simulink library "mbd_s32k1xx_ec_toolbox"  (Simulink 9.0)
settings: Solver=FixedStepDiscrete  StartTime=0.0  StopTime=10.0  FixedStep=0.1  RelTol=1e-3  EnableMultiTasking=on
InitFcn:
  | mbd_s32k_consistency_checks(bdroot(gcs));
(part 3 of 8)

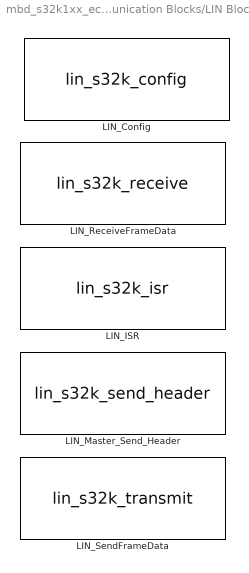
== system mbd_s32k1xx_ec_toolbox/Communication Blocks/LIN Blocks ==
  LIN_Config : S-Function  FunctionName=lin_s32k_config  SFunctionDeploymentMode=off  EnableBusSupport=off  mask(lin_s32k_config){instance=2, baudrate=9600, node_function=MASTER, autobaud_enable=None, rx=PTD6: [LPUART2_RX | Receive], tx=PTD7: [LPUART2_TX | Transmit], cts=PTC12: [LPUART2_CTS | Clear To Send (bar)], rts=PTC13: [LPUART2_RTS | Request To Send]}
      mask prompts: instance "LIN"; baudrate "Baud rate"; node_function "Node function"; autobaud_enable "Autobaud"
      mask help: This block allows to configure LIN module.
      mask init:
      | maskStr = mbd_s32k_lin_config_init();
      | mbd_s32k_lpuart_display_instances(gcb, 'instance');
      | mbd_s32k_lpuart_instance_callback(gcb);
      settings: NameChangeFcn=mbd_s32k_name_check(gcb);
      mask Help: web(fullfile(mbd_s32k_block_help, 'lin', 'lin_config.html'));
      mask TypeOptions instance: 0 | 1 | 2
      mask Callback instance:
      | mbd_s32k_lpuart_instance_callback(gcb);
      | mbd_s32k_lpuart_display_instances(gcb, 'instance');
      mask TypeOptions baudrate: 1200 | 2400 | 4800 | 9600 | 14400 | 19200 | 38400 | 56000 | 57600 | 115200 | 128000 | 256000
      mask TypeOptions node_function: MASTER | SLAVE
      mask TypeOptions autobaud_enable: None | Even | Odd
      mask TypeOptions rx: PTA8: [LPUART2_RX | Receive] | PTA30: [LPUART2_RX | Receive] | PTD6: [LPUART2_RX | Receive] | PTD17: [LPUART2_RX | Receive]
      mask TypeOptions tx: PTA9: [LPUART2_TX | Transmit] | PTA29: [LPUART2_TX | Transmit] | PTD7: [LPUART2_TX | Transmit] | PTE12: [LPUART2_TX | Transmit]
      mask TypeOptions cts: PTC12: [LPUART2_CTS | Clear To Send (bar)] | PTD11: [LPUART2_CTS | Clear To Send (bar)] | PTE9: [LPUART2_CTS | Clear To Send (bar)]
      mask TypeOptions rts: PTC13: [LPUART2_RTS | Request To Send] | PTD12: [LPUART2_RTS | Request To Send] | PTE3: [LPUART2_RTS | Request To Send]
      mask Display:
      | disp(maskStr);
      | image('nxp_logo.png', 'top-right');
  LIN_ISR : S-Function  FunctionName=lin_s32k_isr  Parameters=out_array  SFunctionDeploymentMode=off  EnableBusSupport=off  mask(lin_s32k_isr){instance=2}
      mask prompts: instance "LPUART"
      mask help: This block allows to create receive/transmit ISR routine for the LIN module.
      mask init:
      | mbd_s32k_lpuart_display_instances(gcb, 'instance');
      | [out_struct, out_array] = mbd_s32k_lin_isr_info(gcb);
      | maskStr = mbd_s32k_lin_isr_string();
      settings: NameChangeFcn=mbd_s32k_name_check(gcb);
      mask Help: web(fullfile(mbd_s32k_block_help, 'lin', 'lin_isr.html'));
      mask TypeOptions instance: 0 | 1 | 2
      mask Callback instance: mbd_s32k_lpuart_display_instances(gcb, 'instance');
      mask Display:
      | port_label('output',1,'Trigger')
      | port_label('output',2,'Event')
      | port_label('output',3,'FrameID')
      | disp(maskStr);
      | image('nxp_logo.png', 'top-right');
  LIN_Master_Send_Header : S-Function  FunctionName=lin_s32k_send_header  Parameters=instance  SFunctionDeploymentMode=off  EnableBusSupport=off  mask(lin_s32k_send_header){instance=2}
      mask prompts: instance "LPUART"
      mask help: This block allows to send header [only in master mode].
      mask init:
      | mbd_s32k_lpuart_display_instances(gcb, 'instance');
      settings: NameChangeFcn=mbd_s32k_name_check(gcb);
      mask Help: web(fullfile(mbd_s32k_block_help, 'lin', 'lin_master_send_header.html'));
      mask TypeOptions instance: 0 | 1 | 2
      mask Callback instance: mbd_s32k_lpuart_display_instances(gcb, 'instance');
      mask Display:
      | disp(['LIN ', get_param(gcb, 'instance')]);
      | port_label('input',1,'ID');
      | image('nxp_logo.png', 'top-right');
  LIN_ReceiveFrameData : S-Function  FunctionName=lin_s32k_receive  SFunctionDeploymentMode=off  EnableBusSupport=off  mask(lin_s32k_receive_data){instance=2}
      mask prompts: instance "LIN"
      mask help: This block allows to read data received on LIN bus.
      mask init:
      | mbd_s32k_lpuart_display_instances(gcb, 'instance');
      settings: NameChangeFcn=mbd_s32k_name_check(gcb);
      mask Help: web(fullfile(mbd_s32k_block_help, 'lin', 'lin_receive_frame_data.html'));
      mask TypeOptions instance: 0 | 1 | 2
      mask Callback instance: mbd_s32k_lpuart_display_instances(gcb, 'instance');
      mask Display:
      | disp(['LIN ', get_param(gcb, 'instance')]);
      | port_label('output',1,'data');
      | port_label('input',1,'size');
      | image('nxp_logo.png', 'top-right');
  LIN_SendFrameData : S-Function  FunctionName=lin_s32k_transmit  Parameters=instance  SFunctionDeploymentMode=off  EnableBusSupport=off  mask(lin_s32k_transmit_data){instance=2}
      mask prompts: instance "LPUART"
      mask help: This block allows to transmit data via LIN.
      mask init:
      | mbd_s32k_lpuart_display_instances(gcb, 'instance');
      settings: NameChangeFcn=mbd_s32k_name_check(gcb);
      mask Help: web(fullfile(mbd_s32k_block_help, 'lin', 'lin_send_frame_data.html'));
      mask TypeOptions instance: 0 | 1 | 2
      mask Callback instance: mbd_s32k_lpuart_display_instances(gcb, 'instance');
      mask Display:
      | disp(['LIN ', get_param(gcb, 'instance')]);
      | port_label('input',1,'data');
      | image('nxp_logo.png', 'top-right');

== system mbd_s32k1xx_ec_toolbox/Communication Blocks/SPI Blocks ==
  "LPSPI_Config " : S-Function  FunctionName=lpspi_s32k_config  SFunctionDeploymentMode=off  EnableBusSupport=off  mask(lpspi_s32k_config){InstanceNumber=0, Role=Master, BaudRate=10000, ShowAdvanced=on, sin=PTB3: [LPSPI0_SIN | LPSPI Serial Data Input], sout=PTB1: [LPSPI0_SOUT | LPSPI Serial Data Output], sck=PTB2: [LPSPI0_SCK | LPSPI Serial Clock I/O], pcs0=PTB0: [LPSPI0_PCS0 | Peripheral Chip Select 0], pcs1=PTB5: [LPSPI0_PCS1 | Peripheral Chip Select 1], pcs2=PTE6: [LPSPI0_PCS2 | Peripheral Chip Select 2], pcs3=PTA15: [LPSPI0_PCS3 | Peripheral Chip Select 3], CPHA=0, CPOL=0, BitOrder=MSB first, TransferSize=8, WhichPCS=0, PCSPol=ActiveLow, ContinuousTransfer=off}
      mask prompts: InstanceNumber "Instance"; BaudRate "Baud Rate, bps"; ShowAdvanced "Show advanced options"; BitOrder "Bit order"; TransferSize "Frame size"; WhichPCS "Peripheral CS"; PCSPol "Peripheral CS Polarity"; ContinuousTransfer "Continuous Transfer"
      mask help: This block allows to configure LPSPI module.
      mask init:
      | maskStr = mbd_s32k_lpspi_config_string();
      | mbd_s32k_lpspi_display_instances();
      settings: NameChangeFcn=mbd_s32k_name_check(gcb);
      mask Help: web(fullfile(mbd_s32k_block_help, 'lpspi', 'lpspi_config.html'));
      mask TypeOptions InstanceNumber: 0 | 1 | 2
      mask Callback InstanceNumber:
      | mbd_s32k_lpspi_instance_callback(gcb);
      | mbd_s32k_lpspi_display_instances();
      mask TypeOptions Role: Master | Slave
      mask Callback Role: mbd_s32k_lpspi_config_cbk
      mask Callback ShowAdvanced: mbd_s32k_lpspi_config_cbk()
      mask TypeOptions sin: PTB3: [LPSPI0_SIN | LPSPI Serial Data Input] | PTD16: [LPSPI0_SIN | LPSPI Serial Data Input] | PTE1: [LPSPI0_SIN | LPSPI Serial Data Input]
      mask TypeOptions sout: PTA30: [LPSPI0_SOUT | LPSPI Serial Data Output] | PTB1: [LPSPI0_SOUT | LPSPI Serial Data Output] | PTB4: [LPSPI0_SOUT | LPSPI Serial Data Output] | PTE2: [LPSPI0_SOUT | LPSPI Serial Data Output]
      mask TypeOptions sck: PTB2: [LPSPI0_SCK | LPSPI Serial Clock I/O] | PTC23: [LPSPI0_SCK | LPSPI Serial Clock I/O] | PTD15: [LPSPI0_SCK | LPSPI Serial Clock I/O] | PTE0: [LPSPI0_SCK | LPSPI Serial Clock I/O]
      mask TypeOptions pcs0: None | PTA26: [LPSPI0_PCS0 | Peripheral Chip Select 0] | PTB0: [LPSPI0_PCS0 | Peripheral Chip Select 0] | PTB5: [LPSPI0_PCS0 | Peripheral Chip Select 0]
      mask TypeOptions pcs1: None | PTA31: [LPSPI0_PCS1 | Peripheral Chip Select 1] | PTB5: [LPSPI0_PCS1 | Peripheral Chip Select 1]
      mask TypeOptions pcs2: None | PTE6: [LPSPI0_PCS2 | Peripheral Chip Select 2]
      mask TypeOptions pcs3: None | PTA15: [LPSPI0_PCS3 | Peripheral Chip Select 3]
      mask TypeOptions CPHA: 0 | 1
      mask TypeOptions CPOL: 0 | 1
      mask TypeOptions BitOrder: MSB first | LSB first
      mask TypeOptions WhichPCS: 0 | 1 | 2 | 3
      mask TypeOptions PCSPol: ActiveLow | ActiveHigh
      mask Display:
      | disp(maskStr);
      | image('nxp_logo.png', 'top-right');
  LPSPI_ISR : S-Function  FunctionName=lpspi_s32k_isr  SFunctionDeploymentMode=off  EnableBusSupport=off  mask(lpspi_s32k_isr){instanceNumber=0, isr_lvl=0, role=Master, transfer_end=off, spi_upd=on}
      mask prompts: instanceNumber "Instance"; isr_lvl "ISR Level"; transfer_end "Transfer END"
      mask help: This block allows to create ISR routine (only callback at END OF TRANSFER event) for the LPSPI module.
      mask init:
      | maskStr = mbd_s32k_lpspi_isr_string(gcb);
      settings: NameChangeFcn=mbd_s32k_name_check(gcb);
      mask Help: web(fullfile(mbd_s32k_block_help, 'lpspi', 'lpspi_isr.html'));
      mask TypeOptions instanceNumber: 0 | 1 | 2
      mask TypeOptions isr_lvl: 0 | 1 | 2 | 3 | 4 | 5 | 6 | 7 | 8 | 9 | 10 | 11 | 12 | 13 | 14 | 15
      mask TypeOptions role: Master | Slave
      mask Display:
      | port_label('output',1,'Trigger')
      | disp(maskStr);
      | image('nxp_logo.png', 'top-right');
  LPSPI_Master_Transfer : S-Function  FunctionName=lpspi_s32k_master_transfer  Parameters=instance  SFunctionDeploymentMode=off  EnableBusSupport=off  mask(lpspi_s32k_master_transfer){instance=0, pcs=0, pcs_polarity=ActiveLow, xfermode=Non blocking, timeout=50, spi_upd=on}
      mask prompts: pcs_polarity "PCS Polarity"; xfermode "Transfer mode"
      mask help: Allows to transmit data through a SPI module.
      mask init:
      | maskStr = mbd_s32k_lpspi_master_tx_string(gcb);
      settings: NameChangeFcn=mbd_s32k_name_check(gcb);
      mask Help: web(fullfile(mbd_s32k_block_help, 'lpspi', 'lpspi_master_transfer.html'));
      mask TypeOptions instance: 0 | 1 | 2
      mask TypeOptions pcs: 0 | 1 | 2 | 3
      mask TypeOptions pcs_polarity: ActiveLow | ActiveHigh
      mask TypeOptions xfermode: Blocking | Non blocking
      mask Callback xfermode: mbd_s32k_lpspi_transfer_cbk
      mask Display:
      | port_label('input',1,'Data Tx')
      | port_label('output',1,'Data Rx')
      | disp(maskStr);
      | image('nxp_logo.png', 'top-right');
  LPSPI_Slave_Transfer : S-Function  FunctionName=lpspi_s32k_slave_transfer  Parameters=instance  SFunctionDeploymentMode=off  EnableBusSupport=off  mask(lpspi_s32k_slave_transfer){instance=0, pcs=0, pcs_polarity=ActiveLow, xfermode=Non blocking, timeout=50, spi_upd=on}
      mask prompts: pcs_polarity "PCS Polarity"; xfermode "Transfer mode"
      mask help: Allows to transmit data through a SPI module.
      mask init:
      | maskStr = mbd_s32k_lpspi_master_tx_string(gcb);
      settings: NameChangeFcn=mbd_s32k_name_check(gcb);
      mask Help: web(fullfile(mbd_s32k_block_help, 'lpspi', 'lpspi_slave_transfer.html'));
      mask TypeOptions instance: 0 | 1 | 2
      mask TypeOptions pcs: 0 | 1 | 2 | 3
      mask TypeOptions pcs_polarity: ActiveLow | ActiveHigh
      mask TypeOptions xfermode: Blocking | Non blocking
      mask Callback xfermode: mbd_s32k_lpspi_transfer_cbk
      mask Display:
      | port_label('input',1,'Data Tx')
      | port_label('output',1,'Data Rx')
      | disp(maskStr);
      | image('nxp_logo.png', 'top-right');

== system mbd_s32k1xx_ec_toolbox/Communication Blocks/UART Blocks ==
  LPUART_Config : S-Function  FunctionName=lpuart_s32k_config  SFunctionDeploymentMode=off  EnableBusSupport=off  mask(lpuart_s32k_config){instance=0, baudrate=115200, databits=8, parity=None, sbns=1, bothedge=rising edge, rxinv=off, txinv=off, show_adv_opts=on, brk13=10 - 13 bit times, lbkde=10 - 13 bit times, rx=PTA2: [LPUART0_RX | Receive], tx=PTA3: [LPUART0_TX | Transmit], cts=PTA0: [LPUART0_CTS | Clear To Send (bar)], rts=PTA1: [LPUART0_RTS | Request To Send]}
      mask prompts: instance "LPUART"; baudrate "Baud rate"; databits "Data bits"; parity "Parity mode"; sbns "Stop bit number select"; bothedge "Both edge sampling"; rxinv "Receive data inversion"; txinv "Transmit data inversion"; show_adv_opts "Show advanced options"; brk13 "Transmit break character length"; lbkde "Receive break character detection length"
      mask help: This block allows to configure LPUART module.
      mask init:
      | maskStr = mbd_s32k_lpuart_config_init();
      | mbd_s32k_lpuart_display_instances(gcb, 'instance');
      | mbd_s32k_lpuart_instance_callback(gcb);
      settings: NameChangeFcn=mbd_s32k_name_check(gcb);
      mask Help: web(fullfile(mbd_s32k_block_help, 'lpuart', 'lpuart_config.html'));
      mask TypeOptions instance: 0 | 1 | 2
      mask Callback instance:
      | mbd_s32k_lpuart_instance_callback(gcb);
      | mbd_s32k_lpuart_display_instances(gcb, 'instance');
      mask TypeOptions baudrate: 1200 | 2400 | 4800 | 9600 | 14400 | 19200 | 38400 | 56000 | 57600 | 115200 | 128000 | 256000
      mask TypeOptions databits: 8 | 9 | 10
      mask TypeOptions parity: None | Even | Odd
      mask TypeOptions sbns: 1 | 2
      mask TypeOptions bothedge: rising edge | rising and falling edges
      mask Callback show_adv_opts: mbd_s32k_lpuart_config_cbk()
      mask TypeOptions brk13: 10 - 13 bit times | 13 - 16 bit times
      mask TypeOptions lbkde: 10 - 13 bit times | 13 - 16 bit times
      mask TypeOptions rx: PTA2: [LPUART0_RX | Receive] | PTA28: [LPUART0_RX | Receive] | PTB0: [LPUART0_RX | Receive] | PTC2: [LPUART0_RX | Receive]
      mask TypeOptions tx: PTA3: [LPUART0_TX | Transmit] | PTA27: [LPUART0_TX | Transmit] | PTB1: [LPUART0_TX | Transmit] | PTC3: [LPUART0_TX | Transmit]
      mask TypeOptions cts: PTA0: [LPUART0_CTS | Clear To Send (bar)] | PTC8: [LPUART0_CTS | Clear To Send (bar)]
      mask TypeOptions rts: PTA1: [LPUART0_RTS | Request To Send] | PTC9: [LPUART0_RTS | Request To Send]
      mask Display:
      | image('nxp_logo.png', 'top-right');
      | disp(maskStr);
  LPUART_Receive : S-Function  FunctionName=lpuart_s32k_receive  SFunctionDeploymentMode=off  EnableBusSupport=off  mask(lpuart_s32k_receive){instance=0}
      mask prompts: instance "LPUART"
      mask help: This block allows to read data from LPUART.
      mask init:
      | mbd_s32k_lpuart_display_instances(gcb, 'instance');
      settings: NameChangeFcn=mbd_s32k_name_check(gcb);
      mask Help: web(fullfile(mbd_s32k_block_help, 'lpuart', 'lpuart_receive.html'));
      mask TypeOptions instance: 0 | 1 | 2
      mask Callback instance: mbd_s32k_lpuart_display_instances(gcb, 'instance');
      mask Display:
      | image('nxp_logo.png', 'top-right');
      | disp(['LPUART', get_param(gcb, 'instance')]);
      | port_label('output',1,'data');
      | port_label('input',1,'size');
  LPUART_RxTx_ISR : S-Function  FunctionName=lpuart_s32k_rxtx_isr  Parameters=out_array  SFunctionDeploymentMode=off  EnableBusSupport=off  mask(lpuart_s32k_rxtx_isr){instance=0, prio=0, tie=off, tcie=off, rie=off, ilie=off}
      mask prompts: instance "LPUART"; prio "ISR Priority"; tie "Transmit buffer empty"; tcie "End of transfer"; rie "Receiver buffer full"; ilie "Error event"
      mask help: This block allows to create receive/transmit ISR routine for the LPUART module.
      mask init:
      | mbd_s32k_lpuart_display_instances(gcb, 'instance');
      | [out_struct, out_array] = mbd_s32k_lpuart_isr_info(gcb);
      | maskStr = mbd_s32k_lpuart_isr_string();
      settings: NameChangeFcn=mbd_s32k_name_check(gcb);
      mask Help: web(fullfile(mbd_s32k_block_help, 'lpuart', 'lpuart_rxtx_isr.html'));
      mask TypeOptions instance: 0 | 1 | 2
      mask Callback instance: mbd_s32k_lpuart_display_instances(gcb, 'instance');
      mask TypeOptions prio: 0 | 1 | 2 | 3 | 4 | 5 | 6 | 7 | 8 | 9 | 10 | 11 | 12 | 13 | 14 | 15
      mask Callback prio: mbd_s32k_isr_priority_cbk(gcb, 'prio')
      mask Display:
      | image('nxp_logo.png', 'top-right');
      | port_label('output',1,'Trigger')
      | port_label('output',2,'Status')
      | disp(maskStr);
  LPUART_Transmit : S-Function  FunctionName=lpuart_s32k_transmit  SFunctionDeploymentMode=off  EnableBusSupport=off  mask(lpuart_s32k_transmit){instance=0}
      mask prompts: instance "LPUART"
      mask help: This block allows to transmit data via LPUART.
      mask init:
      | mbd_s32k_lpuart_display_instances(gcb, 'instance');
      settings: NameChangeFcn=mbd_s32k_name_check(gcb);
      mask Help: web(fullfile(mbd_s32k_block_help, 'lpuart', 'lpuart_transmit.html'));
      mask TypeOptions instance: 0 | 1 | 2
      mask Callback instance: mbd_s32k_lpuart_display_instances(gcb, 'instance');
      mask Display:
      | image('nxp_logo.png', 'top-right');
      | disp(['LPUART', get_param(gcb, 'instance')]);
      | port_label('input',1,'data')

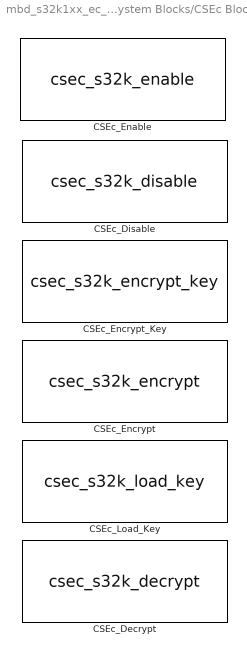
== system mbd_s32k1xx_ec_toolbox/Core and System Blocks/CSEc Blocks ==
  CSEc_Decrypt : S-Function  FunctionName=csec_s32k_decrypt  Parameters=sFuncParams  SFunctionDeploymentMode=off  EnableBusSupport=off  mask(csec_s32k_decrypt){csec_mode=Electronic Codebook (ECB), csec_key_id=RAM_KEY, csec_timeout=1}
      mask prompts: csec_mode "Mode"; csec_key_id "Key ID"; csec_timeout "Timeout (ms)"
      mask help: This block allows to decrypt a cipher text.
      mask init:
      | crlf = sprintf('\n');
      | 
      | mode = get_param(gcb, 'csec_mode');
      | keyId = get_param(gcb, 'csec_key_id');
      | 
      | startIdx = strfind(mode, '(') + 1;
      | endIdx = length(mode) - 1;
      | mode = mode(startIdx:endIdx);
      | 
      | maskStr = [
      |     'CSEc Decrypt' crlf ...
      |     crlf ...
      |     'Mode: ' mode crlf ...
      |     'Key ID: ' keyId crlf];
      | 
      | maskStr = mbd_s32k_csec_init(maskStr);
      | 
      | sFuncParams = uint32([csec_mode])';
      settings: NameChangeFcn=mbd_s32k_name_check(gcb);
      mask Help: web(fullfile(mbd_s32k_block_help, 'csec', 'csec_decrypt.html'));
      mask TypeOptions csec_mode: Electronic Codebook (ECB) | Cipher Block Chaining (CBC)
      mask TypeOptions csec_key_id: RAM_KEY | KEY_1 | KEY_2 | KEY_3 | KEY_4 | KEY_5 | KEY_6 | KEY_7 | KEY_8 | KEY_9 | KEY_10 | KEY_11 | KEY_12 | KEY_13 | KEY_14 | KEY_15 | KEY_16 | KEY_17
      mask Callback csec_timeout: mbd_s32k_csec_decrypt_cbk('csec_timeout');
      mask DialogControl ParametersGroupbox Prompt: Parameters
      mask Display:
      | disp(maskStr);
      | 
      | mode = get_param(gcb, 'csec_mode');
      | 
      | port_label('input', 1, 'Cipher text');
      | if strcmp(mode, 'Cipher Block Chaining (CBC)')
      |     port_label('input', 2, 'IV');
      | end
      | 
      | port_label('output', 1, 'Status');
      | port_label('output', 2, 'Plain text');
      | 
      | image('nxp_logo.png', 'top-right');
  CSEc_Disable : S-Function  FunctionName=csec_s32k_disable  Parameters=sFuncParams  SFunctionDeploymentMode=off  EnableBusSupport=off  mask(csec_s32k_disable){csec_master_key={'0xff', '0xff', '0xff', '0xff', '0xff', '0xff', '0xff', '0xff', '0xff', '0xff', '0xff', '0xff', '0xff', '0xff', '0xff', '0xff'}}
      mask prompts: csec_master_key "Master key"
      mask help: This block allows to disable the CSEc module.
      mask init:
      | maskStr = mbd_s32k_csec_init('CSec Disable');
      | 
      | sFuncParams = uint32([])';
      settings: NameChangeFcn=mbd_s32k_name_check(gcb);
      mask Help: web(fullfile(mbd_s32k_block_help, 'csec', 'csec_disable.html'));
      mask Display:
      | disp(maskStr);
      | port_label('output', 1, 'Status');
      | image('nxp_logo.png', 'top-right');
  CSEc_Enable : S-Function  FunctionName=csec_s32k_enable  Parameters=sFuncParams  SFunctionDeploymentMode=off  EnableBusSupport=off  mask(csec_s32k_enable){csec_num_user_keys=20 keys}
      mask prompts: csec_num_user_keys "User keys"
      mask help: This block allows to enable the CSEc module.
      mask init:
      | maskStr = mbd_s32k_csec_init('CSEc Enable');
      | 
      | sFuncParams = uint32([])';
      settings: NameChangeFcn=mbd_s32k_name_check(gcb);
      mask Help: web(fullfile(mbd_s32k_block_help, 'csec', 'csec_enable.html'));
      mask TypeOptions csec_num_user_keys: Zero | 5 keys | 10 keys | 20 keys
      mask Display:
      | disp(maskStr);
      | image('nxp_logo.png', 'top-right');
  CSEc_Encrypt : S-Function  FunctionName=csec_s32k_encrypt  Parameters=sFuncParams  SFunctionDeploymentMode=off  EnableBusSupport=off  mask(csec_s32k_encrypt){csec_mode=Electronic Codebook (ECB), csec_key_id=RAM_KEY, csec_timeout=1}
      mask prompts: csec_mode "Mode"; csec_key_id "Key ID"; csec_timeout "Timeout (ms)"
      mask help: This block allows to encrypt a plain text.
      mask init:
      | crlf = sprintf('\n');
      | 
      | mode = get_param(gcb, 'csec_mode');
      | keyId = get_param(gcb, 'csec_key_id');
      | 
      | startIdx = strfind(mode, '(') + 1;
      | endIdx = length(mode) - 1;
      | mode = mode(startIdx:endIdx);
      | 
      | 
      | maskStr = [
      |     'CSEc Encrypt' crlf ...
      |     crlf ...
      |     'Mode: ' mode crlf ...
      |     'Key ID: ' keyId crlf];
      | 
      | maskStr = mbd_s32k_csec_init(maskStr);
      | 
      | sFuncParams = uint32([csec_mode])';
      settings: NameChangeFcn=mbd_s32k_name_check(gcb);
      mask Help: web(fullfile(mbd_s32k_block_help, 'csec', 'csec_encrypt.html'));
      mask TypeOptions csec_mode: Electronic Codebook (ECB) | Cipher Block Chaining (CBC)
      mask TypeOptions csec_key_id: RAM_KEY | KEY_1 | KEY_2 | KEY_3 | KEY_4 | KEY_5 | KEY_6 | KEY_7 | KEY_8 | KEY_9 | KEY_10 | KEY_11 | KEY_12 | KEY_13 | KEY_14 | KEY_15 | KEY_16 | KEY_17
      mask Callback csec_timeout: mbd_s32k_csec_encrypt_cbk('csec_timeout');
      mask Display:
      | disp(maskStr);
      | 
      | mode = get_param(gcb, 'csec_mode');
      | 
      | port_label('input', 1, 'Plain text');
      | if strcmp(mode, 'Cipher Block Chaining (CBC)')
      |     port_label('input', 2, 'IV');
      | end
      | 
      | port_label('output', 1, 'Status');
      | port_label('output', 2, 'Cipher text');
      | 
      | image('nxp_logo.png', 'top-right');
  CSEc_Encrypt_Key : S-Function  FunctionName=csec_s32k_encrypt_key  Parameters=[]  SFunctionDeploymentMode=off  EnableBusSupport=off  mask(csec_s32k_encrypt_key){csec_key_id=MASTER_ECU, csec_key={'0xff', '0xff', '0xff', '0xff', '0xff', '0xff', '0xff', '0xff', '0xff', '0xff', '0xff', '0xff', '0xff', '0xff', '0xff', '0xff'}, csec_auth_key_id=MASTER_ECU, csec_auth_key={'0xff', '0xff', '0xff', '0xff', '0xff', '0xff', '0xff', '0xff', '0xff', '0xff', '0xff', '0xff', '0xff', '0xff', '0xff', '0xff'}, csec_counter=1}
      mask prompts: csec_key_id "Key ID"; csec_key "Key"; csec_auth_key_id "Auth key ID"; csec_auth_key "Auth key"; csec_counter "Counter (28 bits)"
      mask help: This block allows to encrypt the key before loading it into CSEc module.
      mask init:
      | crlf = sprintf('\n');
      | 
      | authKeyId = get_param(gcb, 'csec_auth_key_id');
      | keyId = get_param(gcb, 'csec_key_id');
      | 
      | maskStr = [
      |     'CSEc Encrypt Key' crlf ...
      |     crlf ...
      |     'Key ID : ' keyId crlf ...
      |     'Authorization Key ID : ' authKeyId crlf];
      | 
      | maskStr = mbd_s32k_csec_init(maskStr);
      | 
      | sFuncParams = uint32([])';
      settings: NameChangeFcn=mbd_s32k_name_check(gcb);
      mask Help: web(fullfile(mbd_s32k_block_help, 'csec', 'csec_encrypt_key.html'));
      mask TypeOptions csec_key_id: MASTER_ECU | RAM_KEY | KEY_1 | KEY_2 | KEY_3 | KEY_4 | KEY_5 | KEY_6 | KEY_7 | KEY_8 | KEY_9 | KEY_10 | KEY_11 | KEY_12 | KEY_13 | KEY_14 | KEY_15 | KEY_16 | KEY_17
      mask Callback csec_key_id: mbd_s32k_csec_encrypt_key_cbk('csec_key_id');
      mask TypeOptions csec_auth_key_id: MASTER_ECU
      mask Display:
      | disp(maskStr);
      | 
      | port_label('output', 1, 'Status');
      | port_label('output', 2, 'M1');
      | port_label('output', 3, 'M2');
      | port_label('output', 4, 'M3');
      | 
      | image('nxp_logo.png', 'top-right');
  CSEc_Load_Key : S-Function  FunctionName=csec_s32k_load_key  Parameters=sFuncParams  SFunctionDeploymentMode=off  EnableBusSupport=off  mask(csec_s32k_load_key){csec_key_id=MASTER_ECU, csec_load_plain_key=off}
      mask prompts: csec_key_id "Key ID"; csec_load_plain_key "Load plain key"
      mask help: This block allows to load a key.
      mask init:
      | crlf = sprintf('\n');
      | 
      | keyId = get_param(gcb, 'csec_key_id');
      | 
      | maskStr = [
      |     'CSEc Load Key' crlf ...
      |     crlf ...
      |     'Key ID : ' keyId crlf];
      | 
      | maskStr = mbd_s32k_csec_init(maskStr);
      | 
      | if strcmp(keyId, 'RAM_KEY')
      |     loadPlainKey = csec_load_plain_key;
      | else
      |     loadPlainKey = 0;
      | end
      | 
      | sFuncParams = uint32([loadPlainKey])';
      settings: NameChangeFcn=mbd_s32k_name_check(gcb);
      mask Help: web(fullfile(mbd_s32k_block_help, 'csec', 'csec_load_key.html'));
      mask TypeOptions csec_key_id: MASTER_ECU | RAM_KEY | KEY_1 | KEY_2 | KEY_3 | KEY_4 | KEY_5 | KEY_6 | KEY_7 | KEY_8 | KEY_9 | KEY_10 | KEY_11 | KEY_12 | KEY_13 | KEY_14 | KEY_15 | KEY_16 | KEY_17
      mask Callback csec_key_id: mbd_s32k_csec_load_key_cbk('csec_key_id');
      mask Display:
      | disp(maskStr);
      | 
      | keyId = get_param(gcb, 'csec_key_id');
      | loadPlainKey = get_param(gcb, 'csec_load_plain_key');
      | 
      | if strcmp(keyId, 'RAM_KEY') && strcmp(loadPlainKey, 'on')
      |     port_label('input', 1, 'Plain key');
      | else
      |     port_label('input', 1, 'M1');
      |     port_label('input', 2, 'M2');
      |     port_label('input', 3, 'M3');
      | end
      | 
      | port_label('output', 1, 'Status');
      | 
      | image('nxp_logo.png', 'top-right');
